simulink subsystem "rss_BatteryFilterCircuit"  (R2022b)
settings: Solver=VariableStepAuto  StartTime=0.0  StopTime=10.0  RelTol=1e-3
undefined symbols (not defined in the file): cstSplyCrctGrndRstn
libraries: fl_lib x6, ee_lib x1
settings Model: Creator=CAV2OFO  LastModifiedBy=CAV2OFO

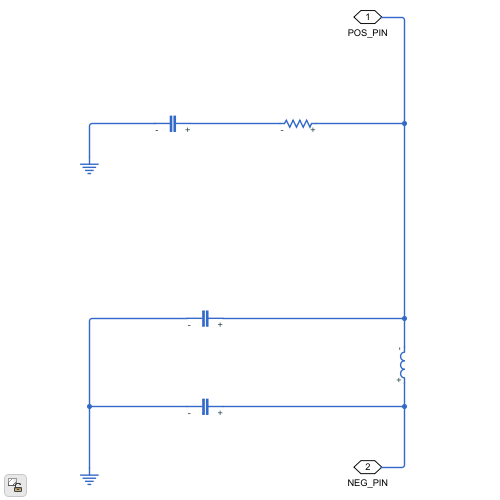
[thumbnail: Simulink's stored preview of the top-level diagram]
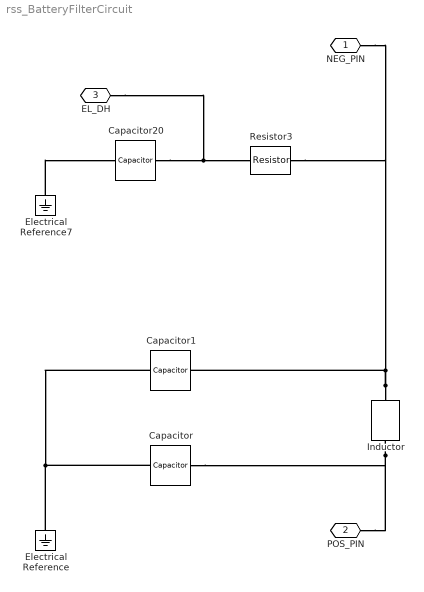
== system rss_BatteryFilterCircuit ==
  Capacitor : fl_lib/Electrical/Electrical Elements/Capacitor  c=cstSplyCrctPosCpct F  r=cstSplyCrctPosCpcrRstn Ohm  g=0 1/Ohm  i_specify=off  i_priority=None  i=0 A  i_nominal_specify=off  i_nominal_unit=A  i_nominal_value=1  v_specify=off  v_priority=None  v=12 V  v_nominal_specify=off  v_nominal_unit=V  v_nominal_value=1  vc_specify=off  vc_priority=High  vc=2 V  vc_nominal_specify=off  vc_nominal_unit=V  vc_nominal_value=1
  Capacitor1 : fl_lib/Electrical/Electrical Elements/Capacitor  c=cstSplyCrctNegCpct F  r=cstSplyCrctNegCpcrRstn Ohm  g=0 1/Ohm  i_specify=off  i_priority=None  i=0 A  i_nominal_specify=off  i_nominal_unit=A  i_nominal_value=1  v_specify=off  v_priority=None  v=12 V  v_nominal_specify=off  v_nominal_unit=V  v_nominal_value=1  vc_specify=off  vc_priority=High  vc=0 V  vc_nominal_specify=off  vc_nominal_unit=V  vc_nominal_value=1
  Capacitor20 : fl_lib/Electrical/Electrical Elements/Capacitor  c=cstSplyCrctGrndCpct F  r=cstSplyCrctGrndCpcrRstn Ohm  g=0 1/Ohm  i_specify=off  i_priority=None  i=0 A  i_nominal_specify=off  i_nominal_unit=A  i_nominal_value=1  v_specify=off  v_priority=None  v=0 V  v_nominal_specify=off  v_nominal_unit=V  v_nominal_value=1  vc_specify=off  vc_priority=High  vc=0 V  vc_nominal_specify=off  vc_nominal_unit=V  vc_nominal_value=1
  Electrical Reference : fl_lib/Electrical/Electrical Elements/Electrical Reference
  Electrical Reference7 : fl_lib/Electrical/Electrical Elements/Electrical Reference
  Inductor : ee_lib/Passive/Inductor  l=cstSplyCrctIndc H  enable_L_tol=0  L_tol=20  tol_distribution=1  nSigma=4  r=cstSplyCrctIndcRstn Ohm  g=0 1/Ohm  enable_operating_limits=0  operating_limit_action=2  max_working_current=1 A  power_rating=1 W  enable_faults=0  fault_action=1  lambdaPercent=50  k_faulted=0.9999  turnsShort=0  openCct=0  groundShort=0  groundShortG=0 1/Ohm  tau_fault=1e-3 s  enable_temporal_fault=0  t_fault=1 s  enable_behavioral_fault=0  max_permissible_voltage=100 V  n_fail_on_voltage=1  max_permissible_current=1 A  t_fail_on_current=1 s  i_L_specify=off  i_L_priority=High  i_L=10 A  i_L_nominal_specify=off  i_L_nominal_unit=A  i_L_nominal_value=1
  Resistor3 : fl_lib/Electrical/Electrical Elements/Resistor  R=cstSplyCrctGrndRstn Ohm  i_specify=off  i_priority=None  i=0 A  i_nominal_specify=off  i_nominal_unit=A  i_nominal_value=1  v_specify=off  v_priority=None  v=0 V  v_nominal_specify=off  v_nominal_unit=V  v_nominal_value=1
  NEG_PIN : PMIOPort  Side=Left
  POS_PIN : PMIOPort  Port=2  Side=Right
  EL_DH : PMIOPort  Port=3  Side=Left
  connections:
  Capacitor1/RConn1 -- Electrical Reference/LConn1 -- Capacitor/RConn1
  Inductor/RConn1 -- NEG_PIN/RConn1 -- Resistor3/LConn1 -- Capacitor1/LConn1
  Inductor/LConn1 -- Capacitor/LConn1 -- POS_PIN/RConn1
  EL_DH/RConn1 -- Capacitor20/LConn1 -- Resistor3/RConn1
  Electrical Reference7/LConn1 -- Capacitor20/RConn1
